simulink model "GoHomeController"  (R2016a)
settings: Solver=ode5  StartTime=0.0  StopTime=100  FixedStep=1/100  RelTol=1e-3  AbsTol=1e-6
model workspace: external: MAT-File GoHomeWorkspace1.mat (data not in the file)
values from neighbouring files (symbols this model uses):
  filtDen = [1 -2.5774735647 5.16845279747 -6.83689517845 7.38438625477 -6.22361169904 4.37103521312 -2.50318155423 1.19677078786 -0.46926551656 0.151337698262 -0.0392326536536 ... (17 elements, 1x17)]    [GoHomeWorkspace.mat]
  filtNum = [9.60149042661e-06 0.000153623846826 0.00115217885119 0.0053768346389 0.0174747125764 0.0419393101834 0.0768887353363 0.10984105048 0.12357118179 0.10984105048 0.0768887353363 0.0419393101834 ... (17 elements, 1x17)]    [GoHomeWorkspace.mat]
  K = [0.865125 0 0 0 0 0.87025 0 0 8 0 0 0 ... (20 elements, 2x10)]    [GoHomeWorkspace.mat]
  Ts = 0.01    [GoHomeWorkspace.mat]
undefined symbols (not defined in the file or in its folder): Crane3D_RangeBit, Crane3D_ScaleCoeff, DiscIntNeverNeededParam
undefined symbols (not defined in the file): RTDAC4PCIBaseAddress
libraries: simulink x1
(part 11 of 11)

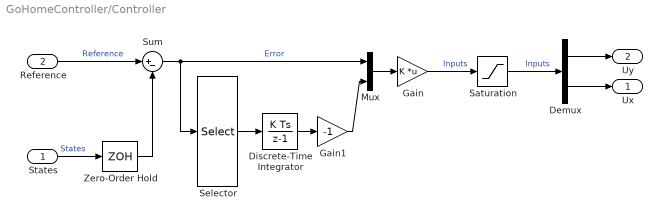
== system GoHomeController/Controller ==
  States : Inport
  Reference : Inport  Port=2
  Demux : Demux  Outputs=2
  Discrete-Time Integrator : DiscreteIntegrator  InitialConditionSetting=State (most efficient)  SampleTime=Ts  ICPrevOutput=DiscIntNeverNeededParam  ICPrevScaledInput=DiscIntNeverNeededParam
  Gain : Gain  Gain=K  Multiplication=Matrix(K*u)
  Gain1 : Gain  Gain=-1
  Mux : Mux  Inputs=2
  Saturation : Saturate  UpperLimit=1  LowerLimit=-1
  Selector : Selector  InputPortWidth=8  IndexOptions=Index vector (dialog)  Indices=[1 3]  OutputSizes=1
  Sum : Sum  Inputs=|+-
  Zero-Order Hold : ZeroOrderHold  SampleTime=Ts
  Ux : Outport
  Uy : Outport  Port=2
  wires:
  States/1 -> Zero-Order Hold/1  "States"
  Reference/1 -> Sum/1  "Reference"
  Saturation/1 -> Demux/1  "Inputs"
  Demux/1 -> Uy/1
  Zero-Order Hold/1 -> Sum/2
  Demux/2 -> Ux/1
  Gain/1 -> Saturation/1  "Inputs"
  Sum/1 -> Mux/1, Selector/1  "Error"
  Selector/1 -> Discrete-Time Integrator/1
  Discrete-Time Integrator/1 -> Gain1/1
  Mux/1 -> Gain/1
  Gain1/1 -> Mux/2

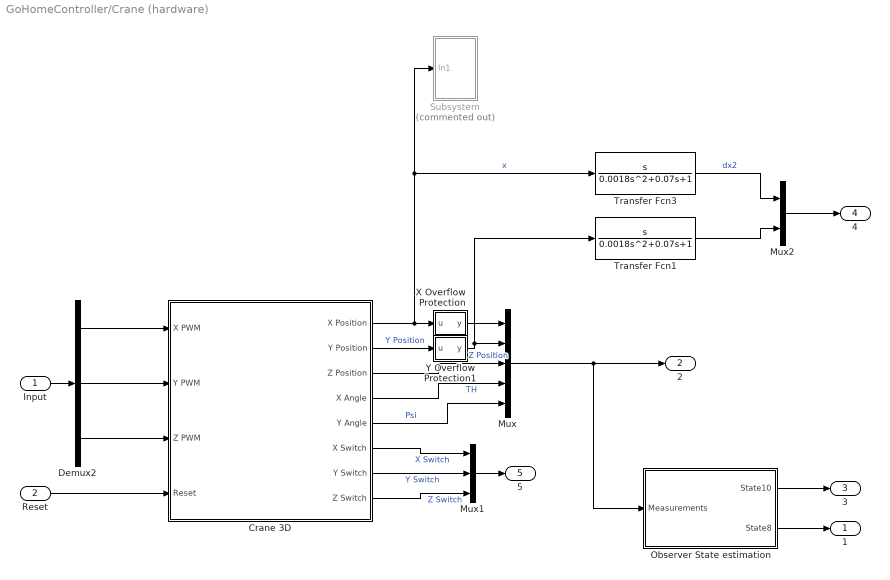
== system GoHomeController/Crane (hardware) ==
  Input : Inport
  Reset : Inport  Port=2
  Crane 3D : Subsystem  mask{BaseAddress=RTDAC4PCIBaseAddress, T0=1/100}
      mask prompts: BaseAddress "Base Address:"; T0 "Sampling Period:"
      mask Display: image(imread('crane.jpeg'))
  Demux2 : Demux  Outputs=3
  Mux : Mux  Inputs=5
  Mux1 : Mux  Inputs=3
  Mux2 : Mux  Inputs=2
  Observer State estimation : Subsystem
  Subsystem : Subsystem  Commented=on
  Transfer Fcn1 : TransferFcn  Numerator=[1 0]  Denominator=[0.0018 0.07 1]
  Transfer Fcn3 : TransferFcn  Numerator=[1 0]  Denominator=[0.0018 0.07 1]
  X Overflow Protection : MATLAB Function  TreatAsAtomicUnit=on
  Y Overflow Protection1 : MATLAB Function  TreatAsAtomicUnit=on
  1 : Outport
  2 : Outport  Port=2
  3 : Outport  Port=3
  4 : Outport  Port=4
  5 : Outport  Port=5
  wires:
  Input/1 -> Demux2/1
  Crane 3D/2(Y Position) -> Y Overflow Protection1/1(u)  "Y Position"
  Crane 3D/3(Z Position) -> Mux/3  "Z Position"
  Crane 3D/4(X Angle) -> Mux/4  "TH"
  Crane 3D/5(Y Angle) -> Mux/5  "Psi"
  Mux/1 -> 2/1, Observer State estimation/1(Measurements)
  Crane 3D/6(X Switch) -> Mux1/1  "X Switch"
  Crane 3D/7(Y Switch) -> Mux1/2  "Y Switch"
  Crane 3D/8(Z Switch) -> Mux1/3  "Z Switch"
  Demux2/1 -> Crane 3D/1(X PWM)
  Demux2/2 -> Crane 3D/2(Y PWM)
  Demux2/3 -> Crane 3D/3(Z PWM)
  Observer State estimation/2(State8) -> 1/1
  Observer State estimation/1(State10) -> 3/1
  Crane 3D/1(X Position) -> Subsystem/1(In1), Transfer Fcn3/1, X Overflow Protection/1(u)  "x"
  Transfer Fcn3/1 -> Mux2/1  "dx2"
  Transfer Fcn1/1 -> Mux2/2
  Mux2/1 -> 4/1
  X Overflow Protection/1(y) -> Mux/1
  Y Overflow Protection1/1(y) -> Transfer Fcn1/1, Mux/2
  Mux1/1 -> 5/1
  Reset/1 -> Crane 3D/4(Reset)

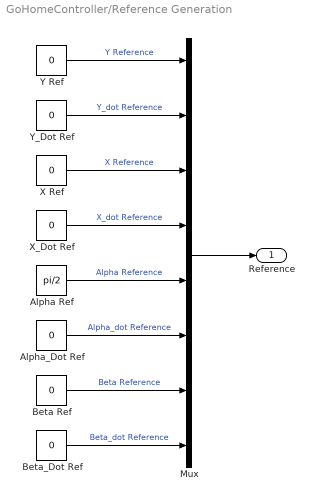
== system GoHomeController/Reference Generation ==
  Alpha Ref : Constant  Value=pi/2
  Alpha_Dot Ref : Constant  Value=0
  Beta Ref : Constant  Value=0
  Beta_Dot Ref : Constant  Value=0
  Mux : Mux  Inputs=8
  X Ref : Constant  Value=0
  X_Dot Ref : Constant  Value=0
  Y Ref : Constant  Value=0
  Y_Dot Ref : Constant  Value=0
  Reference : Outport
  wires:
  Mux/1 -> Reference/1
  Alpha Ref/1 -> Mux/5  "Alpha Reference"
  Alpha_Dot Ref/1 -> Mux/6  "Alpha_dot Reference"
  Beta Ref/1 -> Mux/7  "Beta Reference"
  Beta_Dot Ref/1 -> Mux/8  "Beta_dot Reference"
  X Ref/1 -> Mux/3  "X Reference"
  X_Dot Ref/1 -> Mux/4  "X_dot Reference"
  Y Ref/1 -> Mux/1  "Y Reference"
  Y_Dot Ref/1 -> Mux/2  "Y_dot Reference"

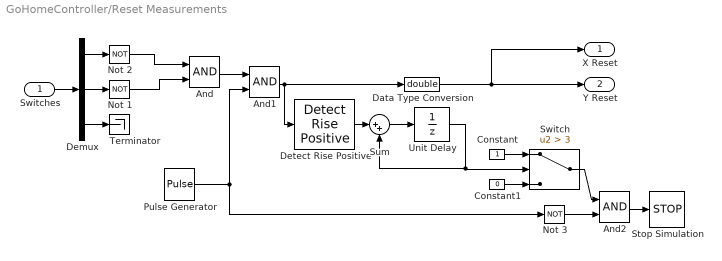
== system GoHomeController/Reset Measurements ==
  Switches : Inport
  And : Logic  AllPortsSameDT=off  OutDataTypeStr=boolean
  And1 : Logic  AllPortsSameDT=off  OutDataTypeStr=boolean
  And2 : Logic  AllPortsSameDT=off  OutDataTypeStr=boolean
  Constant : Constant
  Constant1 : Constant  Value=0
  Data Type Conversion : DataTypeConversion  OutDataTypeStr=double
  Demux : Demux  Outputs=3
  Detect Rise Positive : simulink/Logic and Bit Operations/Detect Rise Positive  vinit=0  OutDataTypeStr=boolean
  Not 1 : Logic  Operator=NOT  AllPortsSameDT=off  OutDataTypeStr=boolean
  Not 2 : Logic  Operator=NOT  AllPortsSameDT=off  OutDataTypeStr=boolean
  Not 3 : Logic  Operator=NOT  AllPortsSameDT=off  OutDataTypeStr=boolean
  Pulse Generator : DiscretePulseGenerator  PulseType=Time based  PulseWidth=50
  Stop Simulation : Stop
  Sum : Sum  Inputs=|++
  Switch : Switch  Criteria=u2 > Threshold  Threshold=3
  Terminator : Terminator
  Unit Delay : UnitDelay  SampleTime=Ts
  X Reset : Outport
  Y Reset : Outport  Port=2
  wires:
  And/1 -> And1/1
  Demux/1 -> Not 2/1
  Demux/2 -> Not 1/1
  Not 1/1 -> And/2
  Not 2/1 -> And/1
  Switches/1 -> Demux/1
  Demux/3 -> Terminator/1
  Pulse Generator/1 -> And1/2, Not 3/1
  And1/1 -> Detect Rise Positive/1, Data Type Conversion/1
  Sum/1 -> Unit Delay/1
  Unit Delay/1 -> Switch/2, Sum/2
  Detect Rise Positive/1 -> Sum/1
  Constant/1 -> Switch/1
  Constant1/1 -> Switch/3
  Data Type Conversion/1 -> Y Reset/1, X Reset/1
  Not 3/1 -> And2/2
  And2/1 -> Stop Simulation/1
  Switch/1 -> And2/1

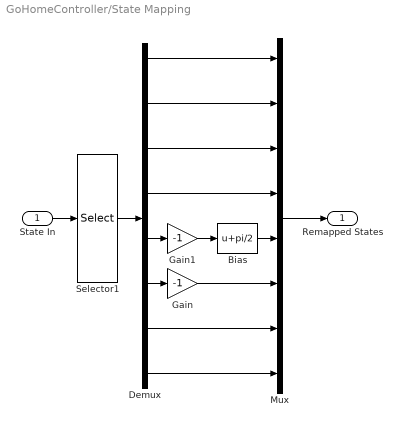
== system GoHomeController/State Mapping ==
  State In : Inport
  Bias : Bias  Bias=pi/2
  Demux : Demux  Outputs=8
  Gain : Gain  Gain=-1
  Gain1 : Gain  Gain=-1
  Mux : Mux  Inputs=8
  Selector1 : Selector  InputPortWidth=8  IndexOptions=Index vector (dialog)  Indices=[3 4 1 2 7 8 5 6]  OutputSizes=1
  Remapped States : Outport
  wires:
  State In/1 -> Selector1/1
  Selector1/1 -> Demux/1
  Demux/7 -> Mux/7
  Demux/8 -> Mux/8
  Demux/6 -> Gain/1
  Demux/5 -> Gain1/1
  Demux/4 -> Mux/4
  Demux/3 -> Mux/3
  Demux/2 -> Mux/2
  Demux/1 -> Mux/1
  Mux/1 -> Remapped States/1
  Gain/1 -> Mux/6
  Gain1/1 -> Bias/1
  Bias/1 -> Mux/5

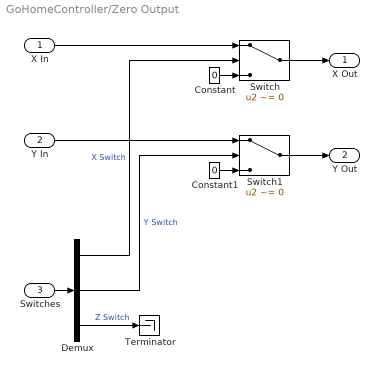
== system GoHomeController/Zero Output ==
  X In : Inport
  Y In : Inport  Port=2
  Switches : Inport  Port=3
  Constant : Constant  Value=0
  Constant1 : Constant  Value=0
  Demux : Demux  Outputs=3
  Switch : Switch  Criteria=u2 ~= 0
  Switch1 : Switch  Criteria=u2 ~= 0
  Terminator : Terminator
  X Out : Outport
  Y Out : Outport  Port=2
  wires:
  Switches/1 -> Demux/1
  X In/1 -> Switch/1
  Constant/1 -> Switch/3
  Demux/1 -> Switch/2  "X Switch"
  Y In/1 -> Switch1/1
  Constant1/1 -> Switch1/3
  Demux/2 -> Switch1/2  "Y Switch"
  Switch/1 -> X Out/1
  Switch1/1 -> Y Out/1
  Demux/3 -> Terminator/1  "Z Switch"

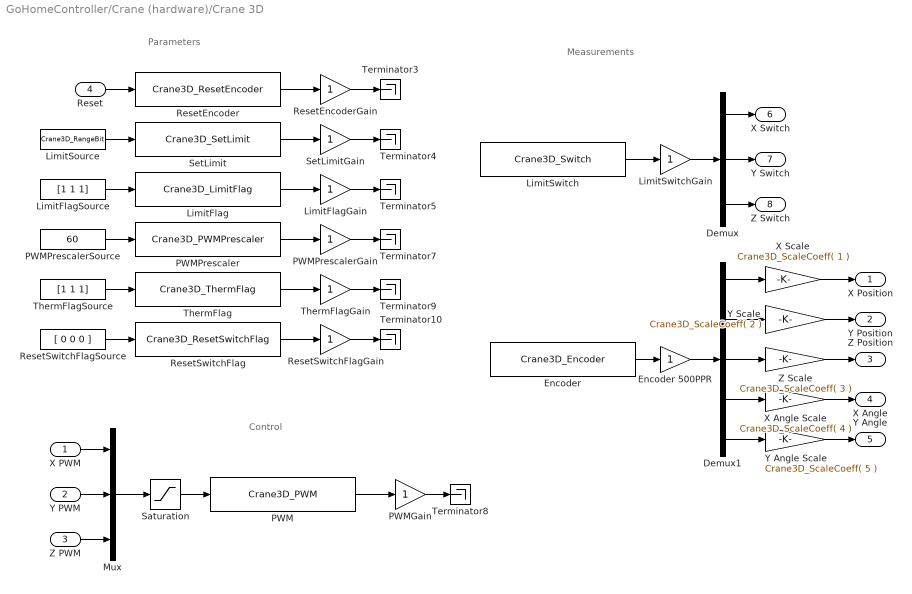
== system GoHomeController/Crane (hardware)/Crane 3D ==
  note: Parameters
  note: Control
  note: Measurements
  X PWM : Inport
  Y PWM : Inport  Port=2
  Z PWM : Inport  Port=3
  Reset : Inport  Port=4
  Demux : Demux  Outputs=3
  Demux1 : Demux  Outputs=5
  Encoder : S-Function  FunctionName=Crane3D_Encoder  Parameters=BaseAddress, T0  SFunctionDeploymentMode=off  EnableBusSupport=off
  Encoder 500PPR : Gain  SaturateOnIntegerOverflow=on  OutDataTypeStr=Inherit: Same as input  ParamDataTypeStr=Inherit: Same as input
  LimitFlag : S-Function  FunctionName=Crane3D_LimitFlag  Parameters=BaseAddress, T0  SFunctionDeploymentMode=off  EnableBusSupport=off
  LimitFlagGain : Gain  SaturateOnIntegerOverflow=on  OutDataTypeStr=Inherit: Same as input  ParamDataTypeStr=Inherit: Same as input
  LimitFlagSource : Constant  Value=[1 1 1]
  LimitSource : Constant  Value=Crane3D_RangeBit
  LimitSwitch : S-Function  FunctionName=Crane3D_Switch  Parameters=BaseAddress, T0  SFunctionDeploymentMode=off  EnableBusSupport=off
  LimitSwitchGain : Gain  SaturateOnIntegerOverflow=on  OutDataTypeStr=Inherit: Same as input  ParamDataTypeStr=Inherit: Same as input
  Mux : Mux  Inputs=3
  PWM : S-Function  FunctionName=Crane3D_PWM  Parameters=BaseAddress, T0  SFunctionDeploymentMode=off  EnableBusSupport=off
  PWMGain : Gain  SaturateOnIntegerOverflow=on  OutDataTypeStr=Inherit: Same as input  ParamDataTypeStr=Inherit: Same as input
  PWMPrescaler : S-Function  FunctionName=Crane3D_PWMPrescaler  Parameters=BaseAddress, T0  SFunctionDeploymentMode=off  EnableBusSupport=off
  PWMPrescalerGain : Gain  SaturateOnIntegerOverflow=on  OutDataTypeStr=Inherit: Same as input  ParamDataTypeStr=Inherit: Same as input
  PWMPrescalerSource : Constant  Value=60
  ResetEncoder : S-Function  FunctionName=Crane3D_ResetEncoder  Parameters=BaseAddress, T0  SFunctionDeploymentMode=off  EnableBusSupport=off
  ResetEncoderGain : Gain  SaturateOnIntegerOverflow=on  OutDataTypeStr=Inherit: Same as input  ParamDataTypeStr=Inherit: Same as input
  "ResetSwitchFlag " : S-Function  FunctionName=Crane3D_ResetSwitchFlag  Parameters=BaseAddress, T0  SFunctionDeploymentMode=off  EnableBusSupport=off
  ResetSwitchFlagGain : Gain  SaturateOnIntegerOverflow=on  OutDataTypeStr=Inherit: Same as input  ParamDataTypeStr=Inherit: Same as input
  ResetSwitchFlagSource : Constant  Value=[ 0 0 0 ]
  Saturation : Saturate  UpperLimit=1  LowerLimit=-1
  SetLimit : S-Function  FunctionName=Crane3D_SetLimit  Parameters=BaseAddress, T0  SFunctionDeploymentMode=off  EnableBusSupport=off
  SetLimitGain : Gain  SaturateOnIntegerOverflow=on  OutDataTypeStr=Inherit: Same as input  ParamDataTypeStr=Inherit: Same as input
  Terminator{3..5,7..10} (7 alike) : Terminator
  "ThermFlag " : S-Function  FunctionName=Crane3D_ThermFlag  Parameters=BaseAddress, T0  SFunctionDeploymentMode=off  EnableBusSupport=off
  ThermFlagGain : Gain  SaturateOnIntegerOverflow=on  OutDataTypeStr=Inherit: Same as input  ParamDataTypeStr=Inherit: Same as input
  ThermFlagSource : Constant  Value=[1 1 1]
  X Angle Scale : Gain  Gain=Crane3D_ScaleCoeff( 4 )  OutDataTypeStr=Inherit: Same as input  ParamDataTypeStr=Inherit: Same as input
  X Scale : Gain  Gain=Crane3D_ScaleCoeff( 1 )  OutDataTypeStr=Inherit: Same as input  ParamDataTypeStr=Inherit: Same as input
  Y Angle Scale : Gain  Gain=Crane3D_ScaleCoeff( 5 )  OutDataTypeStr=Inherit: Same as input  ParamDataTypeStr=Inherit: Same as input
  Y Scale : Gain  Gain=Crane3D_ScaleCoeff( 2 )  OutDataTypeStr=Inherit: Same as input  ParamDataTypeStr=Inherit: Same as input
  Z Scale : Gain  Gain=Crane3D_ScaleCoeff( 3 )  OutDataTypeStr=Inherit: Same as input  ParamDataTypeStr=Inherit: Same as input
  X Position : Outport  InitialOutput=0
  Y Position : Outport  Port=2  InitialOutput=0
  Z Position : Outport  Port=3  InitialOutput=0
  X Angle : Outport  Port=4  InitialOutput=0
  Y Angle : Outport  Port=5  InitialOutput=0
  X Switch : Outport  Port=6  InitialOutput=0
  Y Switch : Outport  Port=7  InitialOutput=0
  Z Switch : Outport  Port=8  InitialOutput=0
  wires:
  Encoder 500PPR/1 -> Demux1/1
  Encoder/1 -> Encoder 500PPR/1
  Saturation/1 -> PWM/1
  Mux/1 -> Saturation/1
  PWM/1 -> PWMGain/1
  PWMGain/1 -> Terminator8/1
  ResetEncoder/1 -> ResetEncoderGain/1
  SetLimit/1 -> SetLimitGain/1
  LimitFlag/1 -> LimitFlagGain/1
  PWMPrescaler/1 -> PWMPrescalerGain/1
  "ThermFlag "/1 -> ThermFlagGain/1
  "ResetSwitchFlag "/1 -> ResetSwitchFlagGain/1
  Reset/1 -> ResetEncoder/1
  LimitSource/1 -> SetLimit/1
  LimitFlagSource/1 -> LimitFlag/1
  PWMPrescalerSource/1 -> PWMPrescaler/1
  ThermFlagSource/1 -> "ThermFlag "/1
  ResetSwitchFlagSource/1 -> "ResetSwitchFlag "/1
  ResetEncoderGain/1 -> Terminator3/1
  SetLimitGain/1 -> Terminator4/1
  LimitFlagGain/1 -> Terminator5/1
  PWMPrescalerGain/1 -> Terminator7/1
  ThermFlagGain/1 -> Terminator9/1
  ResetSwitchFlagGain/1 -> Terminator10/1
  Z PWM/1 -> Mux/3
  Y PWM/1 -> Mux/2
  X PWM/1 -> Mux/1
  LimitSwitch/1 -> LimitSwitchGain/1
  LimitSwitchGain/1 -> Demux/1
  Demux/1 -> X Switch/1
  Demux/2 -> Y Switch/1
  Demux/3 -> Z Switch/1
  Z Scale/1 -> Z Position/1
  X Scale/1 -> X Position/1
  Y Scale/1 -> Y Position/1
  Y Angle Scale/1 -> Y Angle/1
  X Angle Scale/1 -> X Angle/1
  Demux1/5 -> Y Angle Scale/1
  Demux1/4 -> X Angle Scale/1
  Demux1/3 -> Z Scale/1
  Demux1/2 -> Y Scale/1
  Demux1/1 -> X Scale/1

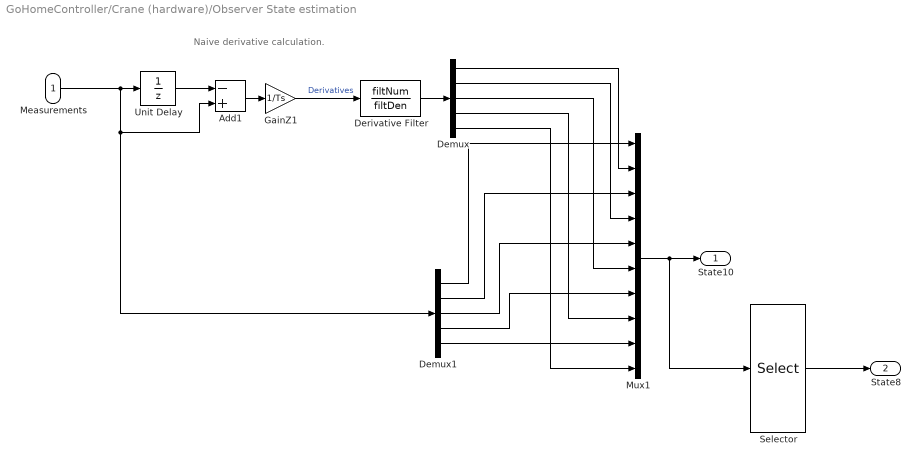
== system GoHomeController/Crane (hardware)/Observer State estimation ==
  note: Naive derivative calculation.
  Measurements : Inport
  Add1 : Sum  Inputs=-+
  Demux : Demux  Outputs=5
  Demux1 : Demux  Outputs=5
  Derivative Filter : DiscreteFilter  Numerator=filtNum  Denominator=filtDen  SampleTime=Ts
  GainZ1 : Gain  Gain=1/Ts  SaturateOnIntegerOverflow=on  OutDataTypeStr=Inherit: Same as input  ParamDataTypeStr=Inherit: Same as input
  Mux1 : Mux  Inputs=10
  Selector : Selector  InputPortWidth=10  IndexOptions=Index vector (dialog)  Indices=[1:4 7:10]  OutputSizes=1
  Unit Delay : UnitDelay  InitialCondition=[0 0 0 0 0]  SampleTime=Ts
  State10 : Outport
  State8 : Outport  Port=2
  wires:
  Unit Delay/1 -> Add1/1
  Add1/1 -> GainZ1/1
  Measurements/1 -> Unit Delay/1, Add1/2, Demux1/1
  GainZ1/1 -> Derivative Filter/1  "Derivatives"
  Mux1/1 -> Selector/1, State10/1
  Demux1/1 -> Mux1/1
  Demux/1 -> Mux1/2
  Demux1/2 -> Mux1/3
  Demux1/3 -> Mux1/5
  Demux1/4 -> Mux1/7
  Demux/2 -> Mux1/4
  Demux/3 -> Mux1/6
  Demux/4 -> Mux1/8
  Selector/1 -> State8/1
  Demux1/5 -> Mux1/9
  Demux/5 -> Mux1/10
  Derivative Filter/1 -> Demux/1

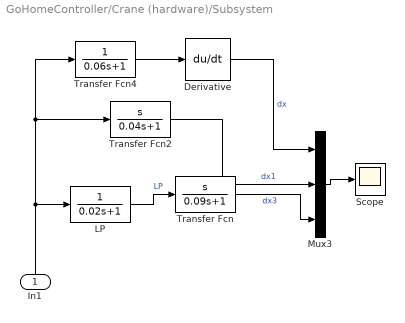
== system GoHomeController/Crane (hardware)/Subsystem ==
  In1 : Inport
  Derivative : Derivative
  LP : TransferFcn  Numerator=[0 1]  Denominator=[0.02 1]
  Mux3 : Mux  Inputs=3
  Scope : Scope
  Transfer Fcn : TransferFcn  Numerator=[1 0]  Denominator=[0.09 1]
  Transfer Fcn2 : TransferFcn  Numerator=[1 0]  Denominator=[0.04 1]
  Transfer Fcn4 : TransferFcn  Numerator=[0 1]  Denominator=[0.06 1]
  wires:
  LP/1 -> Transfer Fcn/1  "LP"
  Transfer Fcn2/1 -> Mux3/2  "dx1"
  Transfer Fcn4/1 -> Derivative/1
  Transfer Fcn/1 -> Mux3/3  "dx3"
  Derivative/1 -> Mux3/1  "dx"
  Mux3/1 -> Scope/1
  In1/1 -> Transfer Fcn4/1, Transfer Fcn2/1, LP/1

== matlab function GoHomeController/Crane (hardware)/Y Overflow Protection1 ==
  data: u input; y output
function y = fcn(u)

y = u;
if (u > 2)
    y = 0;
end

== matlab function GoHomeController/Crane (hardware)/X Overflow Protection ==
  data: u input; y output
function y = fcn(u)

y = u;
if (u > 2)
    y = 0;
end
